simulink model "test_PLECS_V2"  (R2025b)
settings: Solver=VariableStepAuto  StartTime=0.0  StopTime=0.0117  FixedStep=6.5e-6  RelTol=1e-3
undefined symbols (not defined in the file): plecs
libraries: simulink_extras x8, fillib x1
settings Model: Creator=Nelson  LastModifiedBy=llillo
settings RTWCC: GPUComputeCapability=3.5

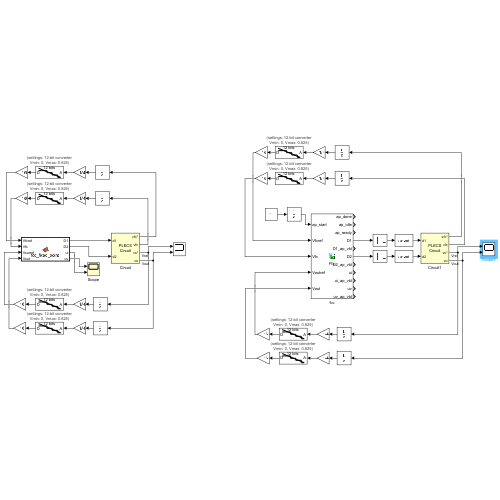
[thumbnail: Simulink's stored preview of the top-level diagram]
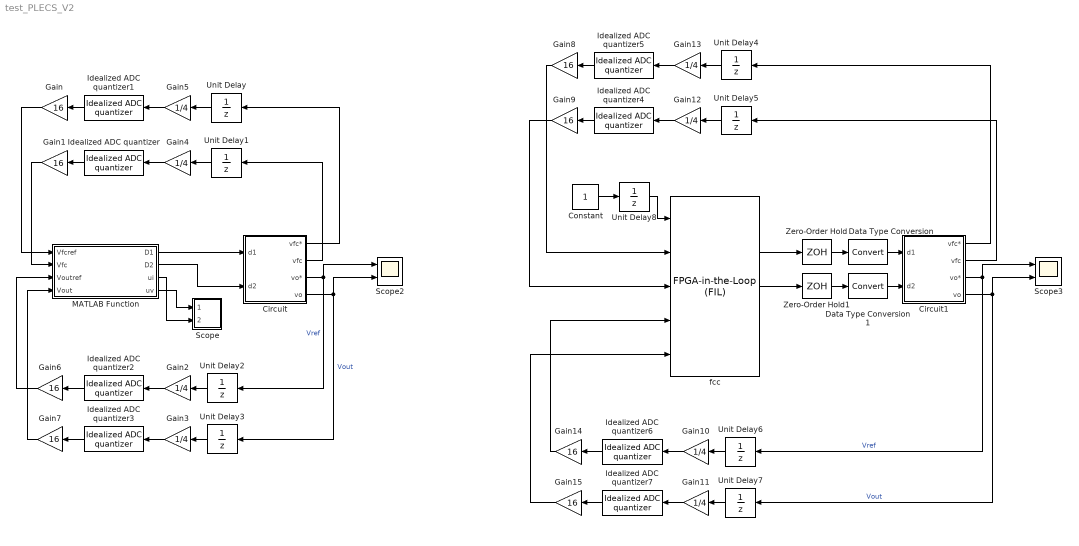
== system test_PLECS_V2 ==
  Circuit : Subsystem  LoadFcn=plecs('sl', 200);  InitFcn=plecs('sl', 214);  StartFcn=plecs('sl', 208);  StopFcn=plecs('sl', 209);  mask(PlecsCircuit){PLECSData=<binary blob, 9016 chars, not shown>}
      mask prompts: PLECSData "PLECS Data (Do not delete or modify!)"
      mask init:
      | % PLACE CUSTOM INITIALIZATIONS ABOVE
      | % DO NOT REMOVE
      | plecs('sl', 215);
      | % DO NOT REMOVE
      settings: CopyFcn=plecs('sl', 203);  DeleteFcn=plecs('sl', 205);  UndoDeleteFcn=plecs('sl', 206);  PreSaveFcn=plecs('sl', 211);  PostSaveFcn=plecs('sl', 201);  NameChangeFcn=plecs('sl', 210);  DestroyFcn=plecs('sl', 207);  PreCopyFcn=plecs('sl', 216);  OpenFcn=plecs('sl', 202);  ErrorFcn=plerrorfcn
      mask Help: eval('plecs(''help'', ''qthelp:///creatingacircuit.html'')')
      mask Display: disp('PLECS\nCircuit')
  Circuit1 : Subsystem  LoadFcn=plecs('sl', 200);  InitFcn=plecs('sl', 214);  StartFcn=plecs('sl', 208);  StopFcn=plecs('sl', 209);  mask(PlecsCircuit){PLECSData=<binary blob, 9016 chars, not shown>}
      mask prompts: PLECSData "PLECS Data (Do not delete or modify!)"
      mask init:
      | % PLACE CUSTOM INITIALIZATIONS ABOVE
      | % DO NOT REMOVE
      | plecs('sl', 215);
      | % DO NOT REMOVE
      settings: CopyFcn=plecs('sl', 203);  DeleteFcn=plecs('sl', 205);  UndoDeleteFcn=plecs('sl', 206);  PreSaveFcn=plecs('sl', 211);  PostSaveFcn=plecs('sl', 201);  NameChangeFcn=plecs('sl', 210);  DestroyFcn=plecs('sl', 207);  PreCopyFcn=plecs('sl', 216);  OpenFcn=plecs('sl', 202);  ErrorFcn=plerrorfcn
      mask Help: eval('plecs(''help'', ''qthelp:///creatingacircuit.html'')')
      mask Display: disp('PLECS\nCircuit')
  Constant : Constant  OutDataTypeStr=boolean
  Data Type Conversion : DataTypeConversion  SaturateOnIntegerOverflow=off  RndMeth=Floor
  Data Type Conversion1 : DataTypeConversion  SaturateOnIntegerOverflow=off  RndMeth=Floor
  Gain{,1,6..9,14..15} (8 alike) : Gain  Gain=16  OutDataTypeStr=uint16  RndMeth=Nearest  SaturateOnIntegerOverflow=on
  Gain{2..5,10..13} (8 alike) : Gain  Gain=1/4
  Idealized ADC quantizer{,1..7} (8 alike) : simulink_extras/Additional Discrete/Idealized ADC quantizer  NumberOfConverterBits=12  Vmin=0  Vmax=0.825  OutputDataType=uint16  OutputNegativeValues=off
  MATLAB Function : MATLAB Function  TreatAsAtomicUnit=on
  Scope : Subsystem  LoadFcn=plecs('sl', 300);  InitFcn=plecs('sl', 314);  StartFcn=plecs('sl', 308);  StopFcn=plecs('sl', 309);  mask{Settings=<binary blob, 900 chars, not shown>}
      mask init:
      | plecs('sl', 315);
      settings: CopyFcn=plecs('sl', 303);  DeleteFcn=plecs('sl', 305);  UndoDeleteFcn=plecs('sl', 306);  PreSaveFcn=plecs('sl', 311);  NameChangeFcn=plecs('sl', 310);  DestroyFcn=plecs('sl', 307);  OpenFcn=plecs('sl', 302);  ErrorFcn=plerrorfcn
      mask Display: plot([0.1 0.9 0.9 0.1 0.1], [0.9 0.9 0.5 0.5 0.9])
  Scope2 : Scope  NumInputPorts=2
      settings: ActiveDisplayYMinimum=-0.2277589913976438  ActiveDisplayYMaximum=2.0498309225787947
  Scope3 : Scope  NumInputPorts=2
      settings: ActiveDisplayYMinimum=-1.094972628574912  ActiveDisplayYMaximum=2.5029972290575895
  Unit Delay{,1..8} (9 alike) : UnitDelay  SampleTime=6.5e-6  HasFrameUpgradeWarning=on
  Zero-Order Hold : ZeroOrderHold  SampleTime=6.5e-6
  Zero-Order Hold1 : ZeroOrderHold  SampleTime=6.5e-6
  fcc : fillib/FPGA-in-the-Loop (FIL)  ForceInterfaceUpdate=0.81472
  wires:
  MATLAB Function/2(D2) -> Circuit/2(d2)
  MATLAB Function/4(uv) -> Scope/1(1)
  MATLAB Function/3(ui) -> Scope/2(2)
  Circuit/1(vfc*) -> Unit Delay/1
  Circuit/2(vfc) -> Unit Delay1/1
  Circuit/3(vo*) -> Unit Delay2/1, Scope2/1  "Vref"
  Circuit/4(vo) -> Scope2/2, Unit Delay3/1  "Vout"
  Unit Delay2/1 -> Gain2/1
  Idealized ADC quantizer1/1 -> Gain/1
  Idealized ADC quantizer/1 -> Gain1/1
  Gain/1 -> MATLAB Function/1(Vfcref)
  Gain1/1 -> MATLAB Function/2(Vfc)
  Idealized ADC quantizer3/1 -> Gain7/1
  Idealized ADC quantizer2/1 -> Gain6/1
  Gain6/1 -> MATLAB Function/3(Voutref)
  Gain2/1 -> Idealized ADC quantizer2/1
  Unit Delay3/1 -> Gain3/1
  Gain3/1 -> Idealized ADC quantizer3/1
  Gain4/1 -> Idealized ADC quantizer/1
  Unit Delay1/1 -> Gain4/1
  Gain5/1 -> Idealized ADC quantizer1/1
  Unit Delay/1 -> Gain5/1
  Gain7/1 -> MATLAB Function/4(Vout)
  MATLAB Function/1(D1) -> Circuit/1(d1)
  Gain8/1 -> fcc/2
  Gain15/1 -> fcc/5
  Gain13/1 -> Idealized ADC quantizer5/1
  Circuit1/3(vo*) -> Unit Delay6/1, Scope3/1  "Vref"
  Gain14/1 -> fcc/4
  Gain9/1 -> fcc/3
  Idealized ADC quantizer6/1 -> Gain14/1
  Idealized ADC quantizer7/1 -> Gain15/1
  Circuit1/2(vfc) -> Unit Delay5/1
  Circuit1/4(vo) -> Scope3/2, Unit Delay7/1  "Vout"
  Gain11/1 -> Idealized ADC quantizer7/1
  Unit Delay4/1 -> Gain13/1
  Circuit1/1(vfc*) -> Unit Delay4/1
  Idealized ADC quantizer5/1 -> Gain8/1
  Unit Delay7/1 -> Gain11/1
  Unit Delay6/1 -> Gain10/1
  Unit Delay5/1 -> Gain12/1
  Gain10/1 -> Idealized ADC quantizer6/1
  Idealized ADC quantizer4/1 -> Gain9/1
  Gain12/1 -> Idealized ADC quantizer4/1
  fcc/4 -> Zero-Order Hold/1
  fcc/6 -> Zero-Order Hold1/1
  Constant/1 -> Unit Delay8/1
  Unit Delay8/1 -> fcc/1
  Zero-Order Hold/1 -> Data Type Conversion/1
  Zero-Order Hold1/1 -> Data Type Conversion1/1
  Data Type Conversion/1 -> Circuit1/1(d1)
  Data Type Conversion1/1 -> Circuit1/2(d2)

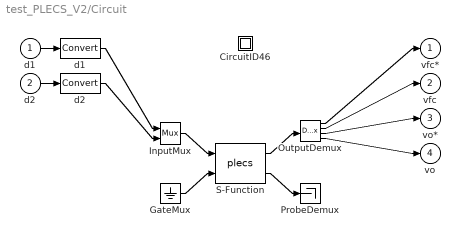
== system test_PLECS_V2/Circuit ==
  d1 : Inport  PortDimensions=1
  d2 : Inport  Port=2  PortDimensions=1
  " CircuitID46 " : Subsystem
  " GateMux " : Ground
  " InputMux " : Mux  Inputs=[ 1 1 ]
  " OutputDemux " : Demux  Outputs=[ 1 1 1 1 ]
  " ProbeDemux " : Terminator
  " S-Function " : S-Function  FunctionName=plecs  SFunctionDeploymentMode=off  EnableBusSupport=off
  " d1 " : DataTypeConversion
  " d2 " : DataTypeConversion
  vfc* : Outport  PortDimensions=1
  vfc : Outport  Port=2  PortDimensions=1
  vo* : Outport  Port=3  PortDimensions=1
  vo : Outport  Port=4  PortDimensions=1
  wires:
  " InputMux "/1 -> " S-Function "/1
  " GateMux "/1 -> " S-Function "/2
  " S-Function "/1 -> " OutputDemux "/1
  " S-Function "/2 -> " ProbeDemux "/1
  d1/1 -> " d1 "/1
  " d1 "/1 -> " InputMux "/1
  d2/1 -> " d2 "/1
  " d2 "/1 -> " InputMux "/2
  " OutputDemux "/1 -> vfc*/1
  " OutputDemux "/2 -> vfc/1
  " OutputDemux "/3 -> vo*/1
  " OutputDemux "/4 -> vo/1

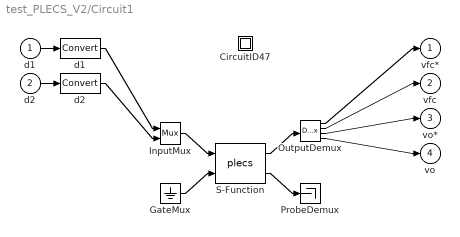
== system test_PLECS_V2/Circuit1 ==
  d1 : Inport  PortDimensions=1
  d2 : Inport  Port=2  PortDimensions=1
  " CircuitID47 " : Subsystem
  " GateMux " : Ground
  " InputMux " : Mux  Inputs=[ 1 1 ]
  " OutputDemux " : Demux  Outputs=[ 1 1 1 1 ]
  " ProbeDemux " : Terminator
  " S-Function " : S-Function  FunctionName=plecs  SFunctionDeploymentMode=off  EnableBusSupport=off
  " d1 " : DataTypeConversion
  " d2 " : DataTypeConversion
  vfc* : Outport  PortDimensions=1
  vfc : Outport  Port=2  PortDimensions=1
  vo* : Outport  Port=3  PortDimensions=1
  vo : Outport  Port=4  PortDimensions=1
  wires:
  " InputMux "/1 -> " S-Function "/1
  " GateMux "/1 -> " S-Function "/2
  " S-Function "/1 -> " OutputDemux "/1
  " S-Function "/2 -> " ProbeDemux "/1
  d1/1 -> " d1 "/1
  " d1 "/1 -> " InputMux "/1
  d2/1 -> " d2 "/1
  " d2 "/1 -> " InputMux "/2
  " OutputDemux "/1 -> vfc*/1
  " OutputDemux "/2 -> vfc/1
  " OutputDemux "/3 -> vo*/1
  " OutputDemux "/4 -> vo/1

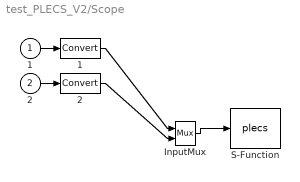
== system test_PLECS_V2/Scope ==
  1 : Inport
  2 : Inport  Port=2
  " 1 " : DataTypeConversion
  " 2 " : DataTypeConversion
  " InputMux " : Mux  Inputs=2
  " S-Function " : S-Function  FunctionName=plecs  SFunctionDeploymentMode=off  EnableBusSupport=off
  wires:
  " InputMux "/1 -> " S-Function "/1
  1/1 -> " 1 "/1
  " 1 "/1 -> " InputMux "/1
  2/1 -> " 2 "/1
  " 2 "/1 -> " InputMux "/2

== system test_PLECS_V2/Circuit/ CircuitID46  ==

== system test_PLECS_V2/Circuit1/ CircuitID47  ==

== matlab function test_PLECS_V2/MATLAB Function ==
  data: Vfcref input; Vfc input; Voutref input; Vout input; D1 output; D2 output; ui output; uv output
%%%%%%%%%%%%%%%%%%%%%%%%%%%%%%%%%%%%%%%%%%%%%%%%%%%%%%%%%%%%%%%%%%%%%%%%%%%%
%                                                                          %
%          Generated by MATLAB 23.2 and Fixed-Point Designer 23.2          %
%                                                                          %
%%%%%%%%%%%%%%%%%%%%%%%%%%%%%%%%%%%%%%%%%%%%%%%%%%%%%%%%%%%%%%%%%%%%%%%%%%%%
function [D1,D2,ui,uv] = fcc_fixed_point(Vfcref,Vfc,Voutref,Vout)
    fm = get_fimath();
    Vfcref_in = fi( Vfcref, 0, 16, 0, fm );
    Vfc_in = fi( Vfc, 0, 16, 0, fm );
    Voutref_in = fi( Voutref, 0, 16, 0, fm );
    Vout_in = fi( Vout, 0, 16, 0, fm );
    [D1_out,D2_out,ui_out,uv_out] = fcc_fixpt( Vfcref_in, Vfc_in, Voutref_in, Vout_in );
    D1 = double( D1_out );
    D2 = double( D2_out );
    ui = double( ui_out );
    uv = double( uv_out );
end

function [D1, D2, ui, uv] = fcc_fixpt(Vfcref, Vfc, Voutref, Vout)
    fm = get_fimath();

    Kpv =  fi(3.214624, 1, 22, 14, fm);
    Kiv = fi(-1.4105, 1, 22, 14, fm);fi(335, 0, 9, 0, fm);
    Kpc =  fi(12.58407884, 1, 22, 14, fm);
    Kic = fi(-12.410690825, 1, 22, 14, fm);
    MAX_DUTY_CYCLE = fi((127), 0, 8, 0, fm);
    gain = fi(4/65535, 1, 22, 14, fm);
    %D1_aux = int8(0);
    %D2_aux = int8(0);

    % Calculo de actuaciones desacopladas
    %ui_aux = int8(0);
    %uv_aux = int8(0);
    ui_aux = fi(pivo_fun(fi(Voutref*gain, 1, 22, 14, fm), fi(Vout*gain, 1, 22, 14, fm), fi(fi(0.0, 0, 1, 0, fm), 1, 22, 14, fm), fi(fi(127.0, 0, 7, 0, fm), 1, 22, 14, fm), fi(Kpv, 1, 22, 14, fm), fi(Kiv, 1, 22, 14, fm)), 1, 22, 14, fm);
    uv_aux = fi(pivf_fun(fi(Vfcref*gain, 1, 22, 14, fm) , fi(Vfc*gain, 1, 22, 14, fm) , fi(fi(-38.0, 1, 7, 0, fm), 1, 22, 14, fm), fi(fi(38.0, 0, 6, 0, fm), 1, 22, 14, fm), fi(Kpc, 1, 22, 14, fm), fi(Kic, 1, 22, 14, fm)), 1, 22, 14, fm);


    D1_aux = fi(fix((ui_aux) + (uv_aux)), 0, 8, 0, fm);
    D2_aux = fi(fix((ui_aux) - (uv_aux)), 0, 8, 0, fm);

    D1 = fi((min(D1_aux, MAX_DUTY_CYCLE)), 0, 8, 0, fm);
    D2 = fi((min(D2_aux, MAX_DUTY_CYCLE)), 0, 8, 0, fm);

    ui = fi((ui_aux), 0, 8, 0, fm);
    uv = fi((uv_aux), 0, 8, 0, fm);
end

%function out = pivf_fun(varargin)
function out = pivo_fun(Vrk, Vk, Vmin, Vmax, Kpid, Kiid)
    % Declarar todas las variables persistentes al inicio
    fm = get_fimath();

    persistent Kp Ki KUi KXi
    persistent xVrk xVk xVmax xVmin xXik xUik xVmk

    % --------------------------
    % Caso: RESET con un solo argumento
    % --------------------------
    %if nargin == 1 && islogical(varargin{1}) && varargin{1} == true
    %    clear pivo_fun
    %    out = 0.0;
    %    return
    %end

    % --------------------------
    % Caso: operación normal
    % --------------------------
    %if nargin ~= 7
    %    error('pivo_fun: Expected 7 input arguments or reset flag.');
    %end

    % Extraer argumentos normalmente
    %Vrk  = varargin{1};
    %Vk   = varargin{2};
    %Vmin = varargin{3};
    %Vmax = varargin{4};
    %Kpid = varargin{5};
    %Kiid = varargin{6};
    %reset = varargin{7}; %#ok<NASGU>  % No se usa ya

    % Inicializar si es primera vez
    if isempty(xXik)
        xXik = fi(zeros(1, 2), 1, 22, 14, fm);
        xUik = fi(zeros(1, 2), 1, 22, 14, fm);
    end

    % Asignación de parámetros
    xVrk = fi(Vrk, 1, 22, 14, fm);
    xVk = fi(Vk, 1, 22, 14, fm);
    xVmax = fi(Vmax, 1, 22, 14, fm);
    xVmin = fi(Vmin, 1, 22, 14, fm);
    Kp = fi(Kpid, 1, 22, 14, fm);
    Ki = fi(Kiid, 1, 22, 14, fm);
    KUi = fi(fi_div(fi_uminus((Kp + Ki)), (Kp * Kpid)), 1, 22, 14, fm);
    KXi = fi(fi_div(fi_uminus(Ki), Kp), 1, 22, 14, fm);

    % PI cálculo
    xXik(2) = xXik(1);
    xUik(2) = xUik(1);
    xXik(1) = KUi * xUik(2) + KXi * xXik(2);
    xUik(1) = Kp * (xVrk - xVk - xXik(1));
    xUik(1) = min(max(xUik(1), xVmin), xVmax);

    xVmk = fi(xUik(1), 1, 22, 14, fm);
    out = fi(xVmk, 1, 22, 14, fm);
end

%function out = pivf_fun(varargin)
function out = pivf_fun(Vrk, Vk, Vmin, Vmax, Kpid, Kiid)
    % Declarar todas las variables persistentes al inicio
    fm = get_fimath();

    persistent Kp Ki KUi KXi
    persistent xVrk xVk xVmax xVmin xXik xUik xVmk

    % --------------------------
    % Caso: RESET con un solo argumento
    % --------------------------
    %if nargin == 1 && islogical(varargin{1}) && varargin{1} == true
    %    clear pivo_fun
    %    out = 0.0;
    %    return
    %end

    % --------------------------
    % Caso: operación normal
    % --------------------------
    %if nargin ~= 7
    %    error('pivo_fun: Expected 7 input arguments or reset flag.');
    %end

    % Extraer argumentos normalmente
    %Vrk  = varargin{1};
    %Vk   = varargin{2};
    %Vmin = varargin{3};
    %Vmax = varargin{4};
    %Kpid = varargin{5};
    %Kiid = varargin{6};
    %reset = varargin{7}; %#ok<NASGU>  % No se usa ya

    % Inicializar si es primera vez
    if isempty(xXik)
        xXik = fi(zeros(1, 2), 1, 22, 14, fm);
        xUik = fi(zeros(1, 2), 1, 22, 14, fm);
    end

    % Asignación de parámetros
    xVrk = fi(Vrk, 1, 22, 14, fm);
    xVk = fi(Vk, 1, 22, 14, fm);
    xVmax = fi(Vmax, 1, 22, 14, fm);
    xVmin = fi(Vmin, 1, 22, 14, fm);
    Kp = fi(Kpid, 1, 22, 14, fm);
    Ki = fi(Kiid, 1, 22, 14, fm);
    KUi = fi(fi_div(fi_uminus((Kp + Ki)), (Kp * Kpid)), 1, 22, 14, fm);
    KXi = fi(fi_div(fi_uminus(Ki), Kp), 1, 22, 14, fm);

    % PI cálculo
    xXik(2) = xXik(1);
    xUik(2) = xUik(1);
    xXik(1) = KUi * xUik(2) + KXi * xXik(2);
    xUik(1) = Kp * (fi_signed(xVrk - xVk) - xXik(1));
    xUik(1) = min(max(xUik(1), xVmin), xVmax);

    xVmk = fi(xUik(1), 1, 22, 14, fm);
    out = fi(xVmk, 1, 22, 14, fm);
end



function ntype = divideType(a,b)
    coder.inline( 'always' );
    nt1 = numerictype( a );
    nt2 = numerictype( b );
    maxFL = max( [ min( nt1.WordLength, nt1.FractionLength ), min( nt2.WordLength, nt2.FractionLength ) ] );
    FL = max( maxFL, 24 );
    extraBits = (FL - maxFL);
    WL = nt1.WordLength + nt2.WordLength;
    WL = min( WL, 124 );
    if (WL + extraBits)<64
        ntype = numerictype( nt1.Signed || nt2.Signed, WL + extraBits, FL );
    else
        ntype = numerictype( nt1.Signed || nt2.Signed, WL, FL );
    end
end


function c = fi_div(a,b)
    coder.inline( 'always' );
    a1 = fi( a, 'RoundMode', 'fix' );
    b1 = fi( b, 'RoundMode', 'fix' );
    nType = divideType( a1, b1 );
    if isfi( a ) && isfi( b ) && isscalar( b )
        c1 = divide( nType, a1, b1 );
        c = fi( c1, numerictype( c1 ), fimath( a ) );
    else
        c = fi( a / b, nType );
    end
end


function y = fi_signed(a)
    coder.inline( 'always' );
    if isfi( a ) && ~(issigned( a ))
        nt = numerictype( a );
        new_nt = numerictype( 1, nt.WordLength + 1, nt.FractionLength );
        y = fi( a, new_nt, fimath( a ) );
    else
        y = a;
    end
end


function y = fi_uminus(a)
    coder.inline( 'always' );
    if isfi( a )
        nt = numerictype( a );
        new_nt = numerictype( 1, nt.WordLength + 1, nt.FractionLength );
        y = -fi( a, new_nt, fimath( a ) );
    else
        y = -a;
    end
end

function fm = get_fimath()
	fm = fimath('RoundingMethod', 'Round',...
	     'OverflowAction', 'Saturate',...
	     'ProductMode','FullPrecision',...
	     'SumMode','FullPrecision');
end
